simulink model "traffic_simulink_model"  (R2023b)
settings: Solver=VariableStepAuto  StartTime=0.0  StopTime=10.0  RelTol=1e-3
settings Model: Creator=agp20009  LastModifiedBy=agp20009

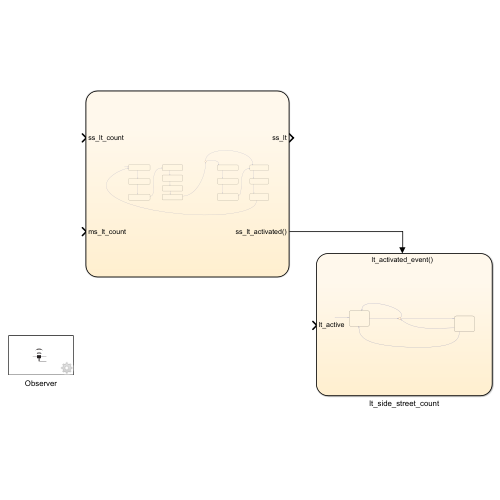
[thumbnail: Simulink's stored preview of the top-level diagram]
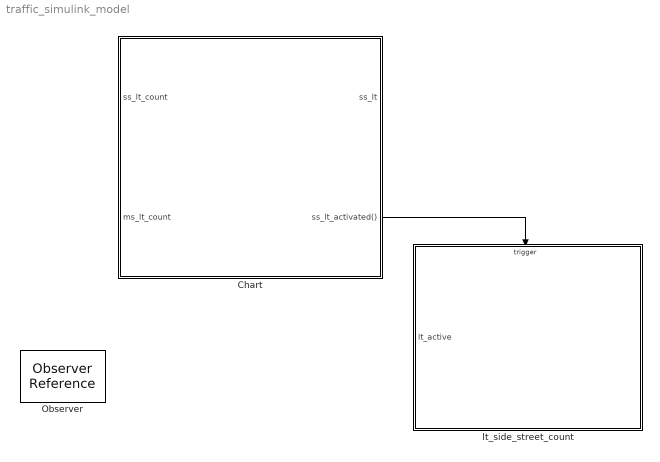
== system traffic_simulink_model ==
  Chart : Stateflow chart  TreatAsAtomicUnit=on
  Observer : ObserverReference  ObserverModelName=Modelling_final_Observer1
  lt_side_street_count : Stateflow chart  TreatAsAtomicUnit=on
  wires:
  Chart/2(ss_lt_activated()) -> lt_side_street_count/Trigger

== stateflow chart traffic_simulink_model/lt_side_street_count ==
  state left_turn_active
    lt_waiting_count=0;
  state lt_cars_queueing
  (junction 3) -> left_turn_active [order 1] : [lt_active]
  (default) -> left_turn_active
  left_turn_active -> (junction 3) : after((15 * rand()) + 5, sec)
  (junction 3) -> lt_cars_queueing [order 2] : [~lt_active]{lt_waiting_count = lt_waiting_count + 1;}
  lt_cars_queueing -> (junction 3) [order 1] : after((15*rand()) + 5, sec)
  lt_cars_queueing -> left_turn_active [order 2] : lt_activated_event
  data: lt_waiting_count local; lt_active input
  events: lt_activated_event input FUNCTION_CALL_EVENT

== stateflow chart traffic_simulink_model/Chart ==
  state main_street_left_turn_initial
    ms_lt=1; ms_gl=0;
    ss_lt=0; ss_gl=0;
  state main_street_green_initial
    ms_lt=0; ms_gl=1;
    ss_lt=0; ss_gl=0;
  state side_street_left_turn_initial
    ms_lt=0; ms_gl=0;
    ss_lt=1; ss_gl=0;
  state side_street_green_initial
    ms_lt=0; ms_gl=0;
    ss_lt=0; ss_gl=1;
  state main_street_green_extendable
    ms_lt=0; ms_gl=1;
    ss_lt=0; ss_gl=0;
  state side_street_left_turn_yellow
    ms_lt=0; ms_gl=0;
    ss_lt=1; ss_gl=0;
  state side_street_yellow
    ms_lt=0; ms_gl=0;
    ss_lt=0; ss_gl=1;
  state main_street_left_turn_yellow
    ms_lt=1; ms_gl=0;
    ss_lt=0; ss_gl=0;
  state main_street_yellow
    ms_lt=0; ms_gl=1;
    ss_lt=0; ss_gl=1;
  state side_street_left_turn_disabled
    ms_lt=0; ms_gl=0;
    ss_lt=0; ss_gl=0;
  state side_street_red
    ms_lt=0; ms_gl=0;
    ss_lt=0; ss_gl=1;
  state main_street_left_turn_disabled
    ms_lt=0; ms_gl=0;
    ss_lt=0; ss_gl=0;
  state main_street_red
    ms_lt=0; ms_gl=0;
    ss_lt=0; ss_gl=0;
  (junction 47) -> side_street_green_initial [order 2] : [ss_lt_count==0;]
  (junction 47) -> side_street_left_turn_initial [order 1] : [ss_lt_count>0;]{ss_lt_activated;}
  main_street_red -> (junction 47) : after(2, sec)
  (default) -> main_street_left_turn_initial
  main_street_left_turn_disabled -> main_street_green_initial : after(2, sec)
  side_street_red -> main_street_left_turn_initial : after(2,sec)
  side_street_left_turn_disabled -> side_street_green_initial : after(2, sec)
  side_street_left_turn_initial -> side_street_left_turn_yellow : after(5, sec)
  side_street_green_initial -> side_street_yellow : after(15, sec)
  main_street_left_turn_initial -> main_street_left_turn_yellow : after(9, sec)
  main_street_green_initial -> main_street_green_extendable : after(20, sec)
  main_street_green_extendable -> main_street_yellow : after(10, sec)
  side_street_yellow -> side_street_red : after(2, sec)
  side_street_left_turn_yellow -> side_street_left_turn_disabled : after(2, sec)
  main_street_left_turn_yellow -> main_street_left_turn_disabled : after(2, sec)
  main_street_yellow -> main_street_red : after(2, sec)
  data: ms_lt local; ms_gl local; ss_gl local; ms_extension local; ss_lt output; ss_lt_count input; ms_lt_count input
  events: ss_lt_activated output FUNCTION_CALL_EVENT
